simulink model "GPS1_Kvaser_R2018a_v3_0719"  (R2018a)
settings: Solver=FixedStepAuto  StartTime=0.0  StopTime=inf  FixedStep=0.02  RelTol=1e-3
undefined symbols (not defined in the file): canChannel
libraries: dspinverses x11, canmsglib x6, canlib x4
(part 2 of 2)

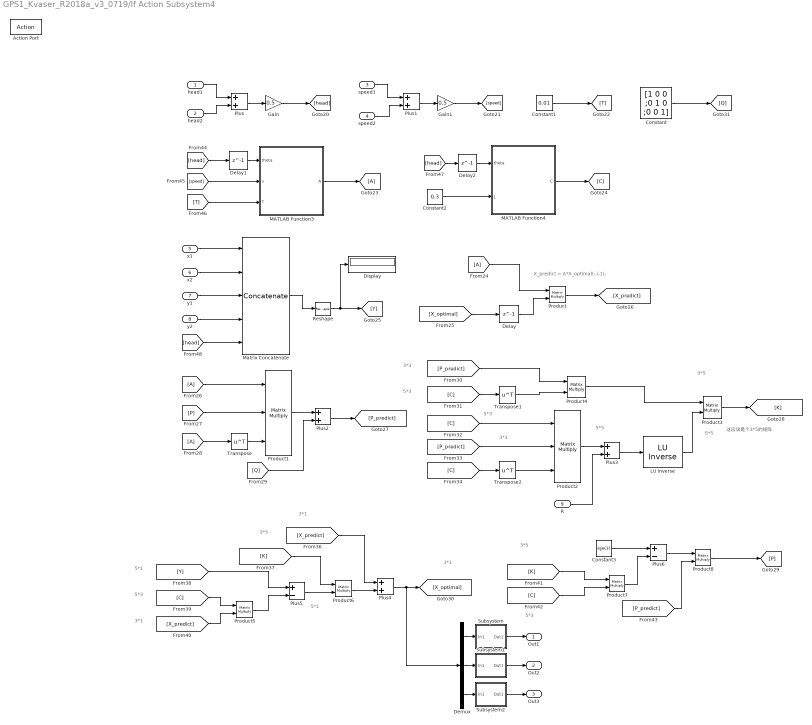
== system GPS1_Kvaser_R2018a_v3_0719/If Action Subsystem4 ==
  note: 5*3
  note: 这应该是个3*5的矩阵
  note: X_predict = A*X_optimal(:,i-1);
  note: 3*1
  note: 5*1
  note: 3*1
  note: 3*5
  note: 5*1
  note: 3*1
  note: 3*5
  note: 5*3
  note: 5*3
  note: 3*3
  note: 5*3
  note: 3*3
  note: 5*5
  note: 5*5
  note: 3*5
  head1 : Inport
  head2 : Inport  Port=2
  speed1 : Inport  Port=3
  speed2 : Inport  Port=4
  x1 : Inport  Port=5
  x2 : Inport  Port=6
  y1 : Inport  Port=7
  y2 : Inport  Port=8
  R : Inport  Port=9
  Action Port : ActionPort
  " LU Inverse" : dspinverses/ LU Inverse
  Constant : Constant  Value=[1 0 0 ;0 1 0 ;0 0 1]
  Constant1 : Constant  Value=0.01
  Constant2 : Constant  Value=0.3
  Constant3 : Constant  Value=eye(3)
  Delay : Delay  DelayLength=1
  Delay1 : Delay  DelayLength=1
  Delay2 : Delay  DelayLength=1
  Demux : Demux  Outputs=3
  Display : Display
  Gain : Gain  Gain=0.5
  Gain1 : Gain  Gain=0.5
  MATLAB Function3 : MATLAB Function  TreatAsAtomicUnit=on
  MATLAB Function4 : MATLAB Function  TreatAsAtomicUnit=on
  Matrix Concatenate : Concatenate  NumInputs=5  Mode=Multidimensional array  ConcatenateDimension=2
  Plus{,1..4} (5 alike) : Sum
  Plus5 : Sum  Inputs=+-
  Plus6 : Sum  Inputs=+-
  Product{,3..8} (7 alike) : Product  Multiplication=Matrix(*)
  Product1 : Product  Inputs=3  Multiplication=Matrix(*)
  Product2 : Product  Inputs=3  Multiplication=Matrix(*)
  Reshape : Reshape  OutputDimensionality=Customize  OutputDimensions=[5,1]
  Subsystem : Subsystem
  Subsystem1 : Subsystem
  Subsystem2 : Subsystem
  Transpose : Math  Operator=transpose  SaturateOnIntegerOverflow=on
  Transpose1 : Math  Operator=transpose  SaturateOnIntegerOverflow=on
  Transpose2 : Math  Operator=transpose  SaturateOnIntegerOverflow=on
  Out1 : Outport
  Out2 : Outport  Port=2
  Out3 : Outport  Port=3
  wires:
  x2/1 -> Matrix Concatenate/2
  y2/1 -> Matrix Concatenate/4
  head1/1 -> Plus/1
  Subsystem2/1(Out1) -> Out3/1
  speed2/1 -> Plus1/2
  x1/1 -> Matrix Concatenate/1
  speed1/1 -> Plus1/1
  head2/1 -> Plus/2
  Demux/1 -> Subsystem/1(In1)
  Demux/3 -> Subsystem2/1(In1)
  [T] -> MATLAB Function3/3(T)
  Product7/1 -> Plus6/2
  Plus/1 -> Gain/1
  [C] -> Product2/1
  [speed] -> MATLAB Function3/2(v)
  Transpose2/1 -> Product2/3
  Reshape/1 -> [Y], Display/1
  Matrix Concatenate/1 -> Reshape/1
  [X_predict] -> Product5/2
  [head] -> Delay2/1
  Transpose/1 -> Product1/3
  Plus1/1 -> Gain1/1
  [P_predict] -> Product4/1
  Gain/1 -> [head]
  Transpose1/1 -> Product4/2
  Constant1/1 -> [T]
  Constant3/1 -> Plus6/1
  " LU Inverse"/1 -> Product3/2
  Product1/1 -> Plus2/1
  [Y] -> Plus5/1
  [A] -> Product/1
  Demux/2 -> Subsystem1/1(In1)
  [K] -> Product7/1
  [A] -> Product1/1
  [Q] -> Plus2/2
  Product2/1 -> Plus3/1
  [head] -> Delay1/1
  [P_predict] -> Product8/2
  [P] -> Product1/2
  [X_predict] -> Plus4/1
  Plus3/1 -> " LU Inverse"/1
  [K] -> Product6/1
  Product3/1 -> [K]
  Plus2/1 -> [P_predict]
  [C] -> Product5/1
  R/1 -> Plus3/2
  Product6/1 -> Plus4/2
  [C] -> Transpose1/1
  [X_optimal] -> Delay/1
  Subsystem1/1(Out1) -> Out2/1
  MATLAB Function4/1(C) -> [C]
  Product5/1 -> Plus5/2
  Product/1 -> [X_predict]
  Product4/1 -> Product3/1
  Plus4/1 -> Demux/1, [X_optimal]
  Constant/1 -> [Q]
  [A] -> Transpose/1
  MATLAB Function3/1(A) -> [A]
  Constant2/1 -> MATLAB Function4/2(L)
  Delay/1 -> Product/2
  Product8/1 -> [P]
  Subsystem/1(Out1) -> Out1/1
  [C] -> Product7/2
  Plus6/1 -> Product8/1
  Plus5/1 -> Product6/2
  y1/1 -> Matrix Concatenate/3
  Gain1/1 -> [speed]
  [head] -> Matrix Concatenate/5
  [C] -> Transpose2/1
  [P_predict] -> Product2/2
  Delay1/1 -> MATLAB Function3/1(theta)
  Delay2/1 -> MATLAB Function4/1(theta)

== system GPS1_Kvaser_R2018a_v3_0719/If Action Subsystem5 ==
  In1 : Inport
  In2 : Inport  Port=2
  In3 : Inport  Port=3
  Action Port : ActionPort
  Out1 : Outport
  Out2 : Outport  Port=2
  Out3 : Outport  Port=3
  wires:
  In1/1 -> Out1/1
  In2/1 -> Out2/1
  In3/1 -> Out3/1

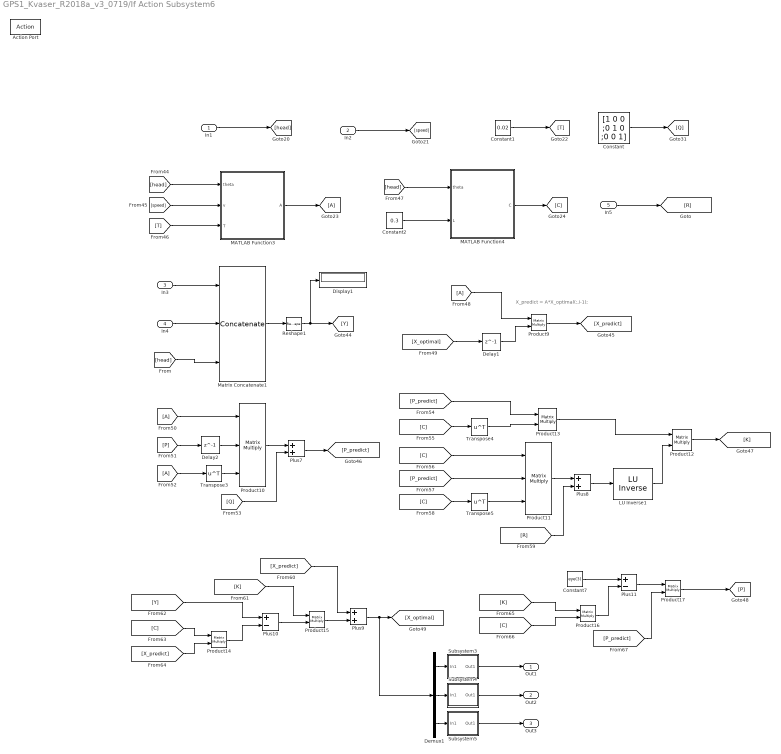
== system GPS1_Kvaser_R2018a_v3_0719/If Action Subsystem6 ==
  note: X_predict = A*X_optimal(:,i-1);
  In1 : Inport
  In2 : Inport  Port=2
  In3 : Inport  Port=3
  In4 : Inport  Port=4
  In5 : Inport  Port=5
  Action Port : ActionPort
  " LU Inverse1" : dspinverses/ LU Inverse
  Constant : Constant  Value=[1 0 0 ;0 1 0 ;0 0 1]
  Constant1 : Constant  Value=0.02
  Constant2 : Constant  Value=0.3
  Constant7 : Constant  Value=eye(3)
  Delay1 : Delay  DelayLength=1
  Delay2 : Delay  DelayLength=1
  Demux1 : Demux  Outputs=3
  Display1 : Display
  MATLAB Function3 : MATLAB Function  TreatAsAtomicUnit=on
  MATLAB Function4 : MATLAB Function  TreatAsAtomicUnit=on
  Matrix Concatenate1 : Concatenate  NumInputs=3  Mode=Multidimensional array  ConcatenateDimension=2
  Plus10 : Sum  Inputs=+-
  Plus11 : Sum  Inputs=+-
  Plus7 : Sum
  Plus8 : Sum
  Plus9 : Sum
  Product10 : Product  Inputs=3  Multiplication=Matrix(*)
  Product11 : Product  Inputs=3  Multiplication=Matrix(*)
  Product{9,12..17} (7 alike) : Product  Multiplication=Matrix(*)
  Reshape1 : Reshape  OutputDimensionality=Customize  OutputDimensions=[3,1]
  Subsystem3 : Subsystem
  Subsystem4 : Subsystem
  Subsystem5 : Subsystem
  Transpose3 : Math  Operator=transpose  SaturateOnIntegerOverflow=on
  Transpose4 : Math  Operator=transpose  SaturateOnIntegerOverflow=on
  Transpose5 : Math  Operator=transpose  SaturateOnIntegerOverflow=on
  Out1 : Outport
  Out2 : Outport  Port=2
  Out3 : Outport  Port=3
  wires:
  [head] -> MATLAB Function4/1(theta)
  Constant1/1 -> [T]
  [speed] -> MATLAB Function3/2(v)
  Subsystem5/1(Out1) -> Out3/1
  [head] -> MATLAB Function3/1(theta)
  Subsystem4/1(Out1) -> Out2/1
  [head] -> Matrix Concatenate1/3
  MATLAB Function3/1(A) -> [A]
  Subsystem3/1(Out1) -> Out1/1
  In4/1 -> Matrix Concatenate1/2
  Product9/1 -> [X_predict]
  [P_predict] -> Product11/2
  [K] -> Product15/1
  Product15/1 -> Plus9/2
  [X_optimal] -> Delay1/1
  [C] -> Product16/2
  Product13/1 -> Product12/1
  Demux1/3 -> Subsystem5/1(In1)
  [C] -> Transpose4/1
  Product12/1 -> [K]
  Transpose3/1 -> Product10/3
  [C] -> Transpose5/1
  [Y] -> Plus10/1
  Product17/1 -> [P]
  Matrix Concatenate1/1 -> Reshape1/1
  [A] -> Transpose3/1
  Transpose4/1 -> Product13/2
  In1/1 -> [head]
  Plus7/1 -> [P_predict]
  [A] -> Product9/1
  In5/1 -> [R]
  [C] -> Product11/1
  Constant2/1 -> MATLAB Function4/2(L)
  MATLAB Function4/1(C) -> [C]
  " LU Inverse1"/1 -> Product12/2
  Transpose5/1 -> Product11/3
  [X_predict] -> Product14/2
  Delay1/1 -> Product9/2
  Plus8/1 -> " LU Inverse1"/1
  [A] -> Product10/1
  Plus10/1 -> Product15/2
  Product11/1 -> Plus8/1
  [K] -> Product16/1
  [R] -> Plus8/2
  [P_predict] -> Product17/2
  [Q] -> Plus7/2
  [P_predict] -> Product13/1
  [C] -> Product14/1
  In2/1 -> [speed]
  Demux1/1 -> Subsystem3/1(In1)
  Reshape1/1 -> [Y], Display1/1
  [X_predict] -> Plus9/1
  Plus9/1 -> Demux1/1, [X_optimal]
  In3/1 -> Matrix Concatenate1/1
  Product14/1 -> Plus10/2
  Constant7/1 -> Plus11/1
  [T] -> MATLAB Function3/3(T)
  Product16/1 -> Plus11/2
  Plus11/1 -> Product17/1
  [P] -> Delay2/1
  Demux1/2 -> Subsystem4/1(In1)
  Constant/1 -> [Q]
  Product10/1 -> Plus7/1
  Delay2/1 -> Product10/2

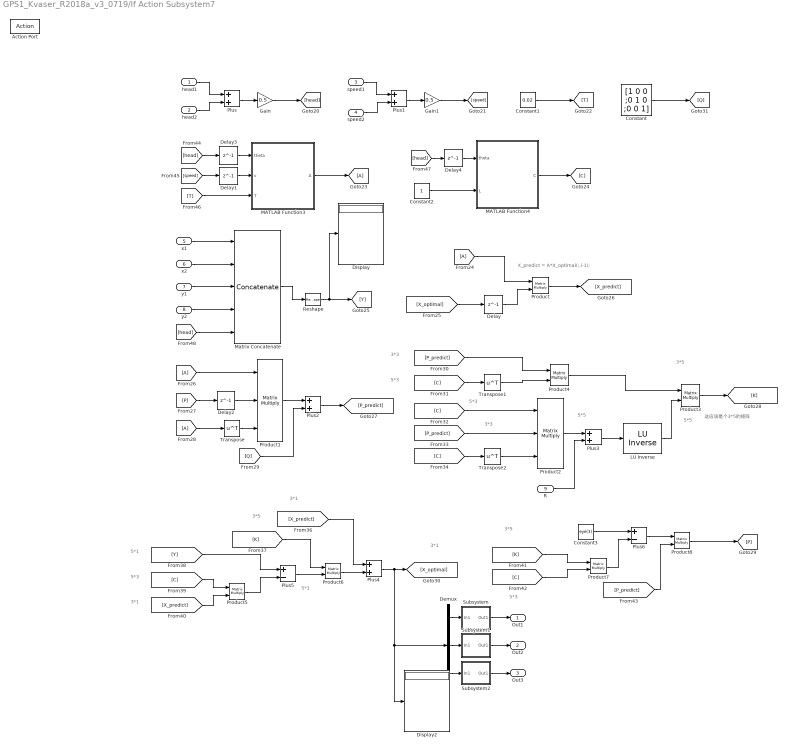
== system GPS1_Kvaser_R2018a_v3_0719/If Action Subsystem7 ==
  note: 5*3
  note: 这应该是个3*5的矩阵
  note: X_predict = A*X_optimal(:,i-1);
  note: 3*1
  note: 5*1
  note: 3*1
  note: 3*5
  note: 5*1
  note: 3*1
  note: 3*5
  note: 5*3
  note: 5*3
  note: 3*3
  note: 5*3
  note: 3*3
  note: 5*5
  note: 5*5
  note: 3*5
  head1 : Inport
  head2 : Inport  Port=2
  speed1 : Inport  Port=3
  speed2 : Inport  Port=4
  x1 : Inport  Port=5
  x2 : Inport  Port=6
  y1 : Inport  Port=7
  y2 : Inport  Port=8
  R : Inport  Port=9
  Action Port : ActionPort
  " LU Inverse" : dspinverses/ LU Inverse
  Constant : Constant  Value=[1 0 0 ;0 1 0 ;0 0 1]
  Constant1 : Constant  Value=0.02
  Constant2 : Constant
  Constant3 : Constant  Value=eye(3)
  Delay{,1..4} (5 alike) : Delay  DelayLength=1
  Demux : Demux  Outputs=3
  Display : Display
  Display2 : Display
  Gain : Gain  Gain=0.5
  Gain1 : Gain  Gain=0.5
  MATLAB Function3 : MATLAB Function  TreatAsAtomicUnit=on
  MATLAB Function4 : MATLAB Function  TreatAsAtomicUnit=on
  Matrix Concatenate : Concatenate  NumInputs=5  Mode=Multidimensional array  ConcatenateDimension=2
  Plus{,1..4} (5 alike) : Sum
  Plus5 : Sum  Inputs=+-
  Plus6 : Sum  Inputs=+-
  Product{,3..8} (7 alike) : Product  Multiplication=Matrix(*)
  Product1 : Product  Inputs=3  Multiplication=Matrix(*)
  Product2 : Product  Inputs=3  Multiplication=Matrix(*)
  Reshape : Reshape  OutputDimensionality=Customize  OutputDimensions=[5,1]
  Subsystem : Subsystem
  Subsystem1 : Subsystem
  Subsystem2 : Subsystem
  Transpose : Math  Operator=transpose  SaturateOnIntegerOverflow=on
  Transpose1 : Math  Operator=transpose  SaturateOnIntegerOverflow=on
  Transpose2 : Math  Operator=transpose  SaturateOnIntegerOverflow=on
  Out1 : Outport
  Out2 : Outport  Port=2
  Out3 : Outport  Port=3
  wires:
  x2/1 -> Matrix Concatenate/2
  y2/1 -> Matrix Concatenate/4
  head1/1 -> Plus/1
  Subsystem2/1(Out1) -> Out3/1
  speed2/1 -> Plus1/2
  x1/1 -> Matrix Concatenate/1
  speed1/1 -> Plus1/1
  head2/1 -> Plus/2
  Demux/1 -> Subsystem/1(In1)
  Demux/3 -> Subsystem2/1(In1)
  [T] -> MATLAB Function3/3(T)
  Product7/1 -> Plus6/2
  Plus/1 -> Gain/1
  [C] -> Product2/1
  [speed] -> Delay1/1
  Transpose2/1 -> Product2/3
  Reshape/1 -> [Y], Display/1
  Matrix Concatenate/1 -> Reshape/1
  [X_predict] -> Product5/2
  Transpose/1 -> Product1/3
  Plus1/1 -> Gain1/1
  [P_predict] -> Product4/1
  Gain/1 -> [head]
  Transpose1/1 -> Product4/2
  Constant1/1 -> [T]
  Constant3/1 -> Plus6/1
  " LU Inverse"/1 -> Product3/2
  Product1/1 -> Plus2/1
  [Y] -> Plus5/1
  [A] -> Product/1
  Demux/2 -> Subsystem1/1(In1)
  [K] -> Product7/1
  [A] -> Product1/1
  [Q] -> Plus2/2
  Product2/1 -> Plus3/1
  [P_predict] -> Product8/2
  [X_predict] -> Plus4/1
  Plus3/1 -> " LU Inverse"/1
  [K] -> Product6/1
  Product3/1 -> [K]
  Plus2/1 -> [P_predict]
  [C] -> Product5/1
  R/1 -> Plus3/2
  Product6/1 -> Plus4/2
  [C] -> Transpose1/1
  [X_optimal] -> Delay/1
  Subsystem1/1(Out1) -> Out2/1
  MATLAB Function4/1(C) -> [C]
  Product5/1 -> Plus5/2
  Product/1 -> [X_predict]
  Product4/1 -> Product3/1
  Plus4/1 -> Display2/1, Demux/1, [X_optimal]
  Constant/1 -> [Q]
  [A] -> Transpose/1
  MATLAB Function3/1(A) -> [A]
  Constant2/1 -> MATLAB Function4/2(L)
  Delay/1 -> Product/2
  Product8/1 -> [P]
  Subsystem/1(Out1) -> Out1/1
  [C] -> Product7/2
  Plus6/1 -> Product8/1
  Plus5/1 -> Product6/2
  y1/1 -> Matrix Concatenate/3
  Gain1/1 -> [speed]
  [head] -> Matrix Concatenate/5
  [C] -> Transpose2/1
  [P_predict] -> Product2/2
  [head] -> Delay3/1
  [head] -> Delay4/1
  [P] -> Delay2/1
  Delay1/1 -> MATLAB Function3/2(v)
  Delay3/1 -> MATLAB Function3/1(theta)
  Delay4/1 -> MATLAB Function4/1(theta)
  Delay2/1 -> Product1/2

== system GPS1_Kvaser_R2018a_v3_0719/If Action Subsystem8 ==
  In1 : Inport
  In2 : Inport  Port=2
  In3 : Inport  Port=3
  Action Port : ActionPort
  Out1 : Outport
  Out2 : Outport  Port=2
  Out3 : Outport  Port=3
  wires:
  In1/1 -> Out1/1
  In2/1 -> Out2/1
  In3/1 -> Out3/1

== system GPS1_Kvaser_R2018a_v3_0719/Subsystem ==
  In1 : Inport
  Delay : Delay  DelayLength=1
  Gain : Gain  Gain=0.1
  Gain1 : Gain  Gain=0.9
  Plus : Sum
  Out1 : Outport
  wires:
  In1/1 -> Gain/1
  Gain/1 -> Plus/1
  Plus/1 -> Delay/1, Out1/1
  Delay/1 -> Gain1/1
  Gain1/1 -> Plus/2

== system GPS1_Kvaser_R2018a_v3_0719/Subsystem1 ==
  In1 : Inport
  Delay : Delay  DelayLength=1
  Gain : Gain  Gain=0.1
  Gain1 : Gain  Gain=0.9
  Plus : Sum
  Out1 : Outport
  wires:
  Gain1/1 -> Plus/2
  Delay/1 -> Gain1/1
  Plus/1 -> Out1/1, Delay/1
  Gain/1 -> Plus/1
  In1/1 -> Gain/1

== system GPS1_Kvaser_R2018a_v3_0719/Subsystem2 ==
  In1 : Inport
  Delay : Delay  DelayLength=1
  Gain : Gain  Gain=0.1
  Gain1 : Gain  Gain=0.9
  Plus : Sum
  Out1 : Outport
  wires:
  In1/1 -> Gain/1
  Gain/1 -> Plus/1
  Plus/1 -> Delay/1, Out1/1
  Delay/1 -> Gain1/1
  Gain1/1 -> Plus/2

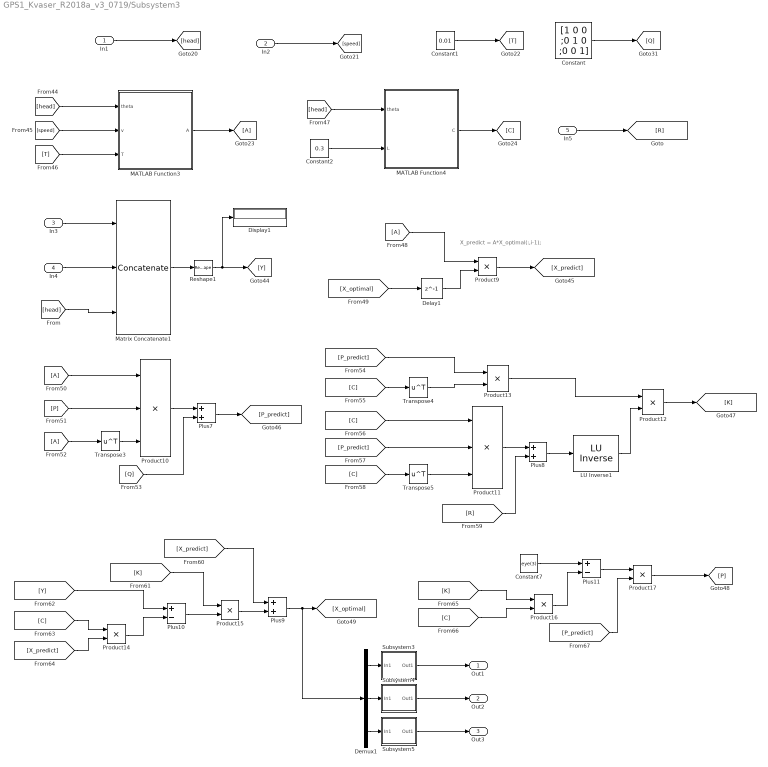
== system GPS1_Kvaser_R2018a_v3_0719/Subsystem3 ==
  note: X_predict = A*X_optimal(:,i-1);
  In1 : Inport
  In2 : Inport  Port=2
  In3 : Inport  Port=3
  In4 : Inport  Port=4
  In5 : Inport  Port=5
  " LU Inverse1" : dspinverses/ LU Inverse
  Constant : Constant  Value=[1 0 0 ;0 1 0 ;0 0 1]
  Constant1 : Constant  Value=0.01
  Constant2 : Constant  Value=0.3
  Constant7 : Constant  Value=eye(3)
  Delay1 : Delay  DelayLength=1
  Demux1 : Demux  Outputs=3
  Display1 : Display
  MATLAB Function3 : MATLAB Function  TreatAsAtomicUnit=on
  MATLAB Function4 : MATLAB Function  TreatAsAtomicUnit=on
  Matrix Concatenate1 : Concatenate  NumInputs=3  Mode=Multidimensional array  ConcatenateDimension=2
  Plus10 : Sum  Inputs=+-
  Plus11 : Sum  Inputs=+-
  Plus7 : Sum
  Plus8 : Sum
  Plus9 : Sum
  Product10 : Product  Inputs=3
  Product11 : Product  Inputs=3
  Product{9,12..17} (7 alike) : Product
  Reshape1 : Reshape  OutputDimensionality=Customize  OutputDimensions=[3,1]
  Subsystem3 : Subsystem
  Subsystem4 : Subsystem
  Subsystem5 : Subsystem
  Transpose3 : Math  Operator=transpose  SaturateOnIntegerOverflow=on
  Transpose4 : Math  Operator=transpose  SaturateOnIntegerOverflow=on
  Transpose5 : Math  Operator=transpose  SaturateOnIntegerOverflow=on
  Out1 : Outport
  Out2 : Outport  Port=2
  Out3 : Outport  Port=3
  wires:
  Product12/1 -> [K]
  [Y] -> Plus10/1
  Product17/1 -> [P]
  Transpose3/1 -> Product10/3
  [C] -> Transpose5/1
  Demux1/3 -> Subsystem5/1(In1)
  Product13/1 -> Product12/1
  Demux1/2 -> Subsystem4/1(In1)
  [C] -> Transpose4/1
  Plus10/1 -> Product15/2
  [C] -> Product16/2
  [X_optimal] -> Delay1/1
  [R] -> Plus8/2
  [P_predict] -> Product11/2
  Product9/1 -> [X_predict]
  [K] -> Product15/1
  Product15/1 -> Plus9/2
  Product10/1 -> Plus7/1
  Plus11/1 -> Product17/1
  [P] -> Product10/2
  Product16/1 -> Plus11/2
  Product14/1 -> Plus10/2
  Plus9/1 -> Demux1/1, [X_optimal]
  [X_predict] -> Plus9/1
  [C] -> Product14/1
  Demux1/1 -> Subsystem3/1(In1)
  Subsystem3/1(Out1) -> Out1/1
  Reshape1/1 -> [Y], Display1/1
  Subsystem5/1(Out1) -> Out3/1
  [P_predict] -> Product13/1
  [Q] -> Plus7/2
  Subsystem4/1(Out1) -> Out2/1
  [P_predict] -> Product17/2
  Product11/1 -> Plus8/1
  [K] -> Product16/1
  [A] -> Product10/1
  Constant7/1 -> Plus11/1
  Plus8/1 -> " LU Inverse1"/1
  Delay1/1 -> Product9/2
  [X_predict] -> Product14/2
  " LU Inverse1"/1 -> Product12/2
  Transpose5/1 -> Product11/3
  Transpose4/1 -> Product13/2
  Plus7/1 -> [P_predict]
  Matrix Concatenate1/1 -> Reshape1/1
  [C] -> Product11/1
  [A] -> Transpose3/1
  [A] -> Product9/1
  [T] -> MATLAB Function3/3(T)
  MATLAB Function3/1(A) -> [A]
  Constant/1 -> [Q]
  Constant2/1 -> MATLAB Function4/2(L)
  [head] -> MATLAB Function3/1(theta)
  [speed] -> MATLAB Function3/2(v)
  Constant1/1 -> [T]
  MATLAB Function4/1(C) -> [C]
  [head] -> MATLAB Function4/1(theta)
  In2/1 -> [speed]
  In1/1 -> [head]
  In4/1 -> Matrix Concatenate1/2
  In3/1 -> Matrix Concatenate1/1
  [head] -> Matrix Concatenate1/3
  In5/1 -> [R]

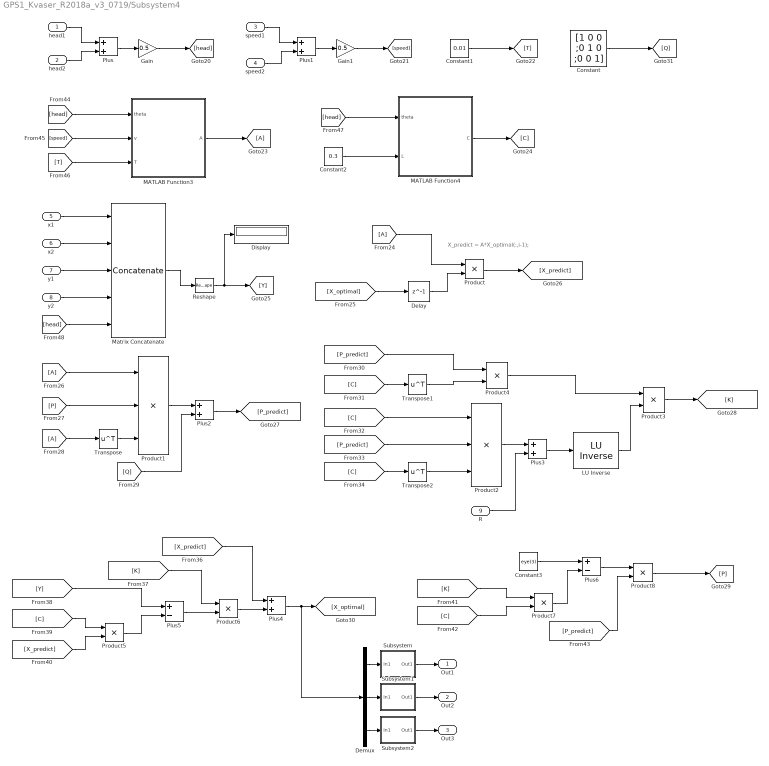
== system GPS1_Kvaser_R2018a_v3_0719/Subsystem4 ==
  note: X_predict = A*X_optimal(:,i-1);
  head1 : Inport
  head2 : Inport  Port=2
  speed1 : Inport  Port=3
  speed2 : Inport  Port=4
  x1 : Inport  Port=5
  x2 : Inport  Port=6
  y1 : Inport  Port=7
  y2 : Inport  Port=8
  R : Inport  Port=9
  " LU Inverse" : dspinverses/ LU Inverse
  Constant : Constant  Value=[1 0 0 ;0 1 0 ;0 0 1]
  Constant1 : Constant  Value=0.01
  Constant2 : Constant  Value=0.3
  Constant3 : Constant  Value=eye(3)
  Delay : Delay  DelayLength=1
  Demux : Demux  Outputs=3
  Display : Display
  Gain : Gain  Gain=0.5
  Gain1 : Gain  Gain=0.5
  MATLAB Function3 : MATLAB Function  TreatAsAtomicUnit=on
  MATLAB Function4 : MATLAB Function  TreatAsAtomicUnit=on
  Matrix Concatenate : Concatenate  NumInputs=5  Mode=Multidimensional array  ConcatenateDimension=2
  Plus{,1..4} (5 alike) : Sum
  Plus5 : Sum  Inputs=+-
  Plus6 : Sum  Inputs=+-
  Product{,3..8} (7 alike) : Product
  Product1 : Product  Inputs=3
  Product2 : Product  Inputs=3
  Reshape : Reshape  OutputDimensionality=Customize  OutputDimensions=[4,1]
  Subsystem : Subsystem
  Subsystem1 : Subsystem
  Subsystem2 : Subsystem
  Transpose : Math  Operator=transpose  SaturateOnIntegerOverflow=on
  Transpose1 : Math  Operator=transpose  SaturateOnIntegerOverflow=on
  Transpose2 : Math  Operator=transpose  SaturateOnIntegerOverflow=on
  Out1 : Outport
  Out2 : Outport  Port=2
  Out3 : Outport  Port=3
  wires:
  Subsystem1/1(Out1) -> Out2/1
  Subsystem/1(Out1) -> Out1/1
  [head] -> Matrix Concatenate/5
  Demux/1 -> Subsystem/1(In1)
  Demux/3 -> Subsystem2/1(In1)
  Demux/2 -> Subsystem1/1(In1)
  [T] -> MATLAB Function3/3(T)
  MATLAB Function4/1(C) -> [C]
  MATLAB Function3/1(A) -> [A]
  Constant/1 -> [Q]
  Constant2/1 -> MATLAB Function4/2(L)
  Product8/1 -> [P]
  [C] -> Transpose2/1
  Plus6/1 -> Product8/1
  [C] -> Product7/2
  Product4/1 -> Product3/1
  Product3/1 -> [K]
  Plus4/1 -> Demux/1, [X_optimal]
  [C] -> Product5/1
  [K] -> Product6/1
  [X_predict] -> Plus4/1
  [X_optimal] -> Delay/1
  Product6/1 -> Plus4/2
  head1/1 -> Plus/1
  [Y] -> Plus5/1
  Product1/1 -> Plus2/1
  [P_predict] -> Product8/2
  [P] -> Product1/2
  [Q] -> Plus2/2
  Product2/1 -> Plus3/1
  [K] -> Product7/1
  speed1/1 -> Plus1/1
  [P_predict] -> Product2/2
  speed2/1 -> Plus1/2
  y2/1 -> Matrix Concatenate/4
  R/1 -> Plus3/2
  Plus3/1 -> " LU Inverse"/1
  " LU Inverse"/1 -> Product3/2
  Constant3/1 -> Plus6/1
  x2/1 -> Matrix Concatenate/2
  [A] -> Product1/1
  Subsystem2/1(Out1) -> Out3/1
  Transpose/1 -> Product1/3
  [P_predict] -> Product4/1
  Transpose1/1 -> Product4/2
  Delay/1 -> Product/2
  Constant1/1 -> [T]
  y1/1 -> Matrix Concatenate/3
  [C] -> Transpose1/1
  Plus2/1 -> [P_predict]
  head2/1 -> Plus/2
  [C] -> Product2/1
  Transpose2/1 -> Product2/3
  [speed] -> MATLAB Function3/2(v)
  Gain1/1 -> [speed]
  Plus1/1 -> Gain1/1
  [X_predict] -> Product5/2
  Matrix Concatenate/1 -> Reshape/1
  Product5/1 -> Plus5/2
  Product7/1 -> Plus6/2
  Product/1 -> [X_predict]
  [A] -> Product/1
  Gain/1 -> [head]
  x1/1 -> Matrix Concatenate/1
  [A] -> Transpose/1
  [head] -> MATLAB Function3/1(theta)
  [head] -> MATLAB Function4/1(theta)
  Plus/1 -> Gain/1
  Reshape/1 -> [Y], Display/1
  Plus5/1 -> Product6/2

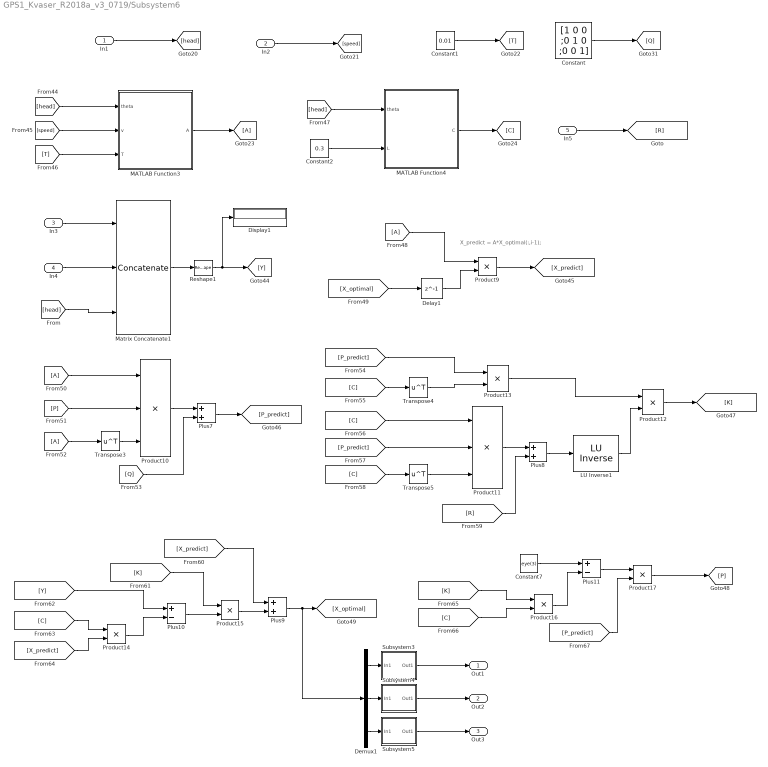
== system GPS1_Kvaser_R2018a_v3_0719/Subsystem6 ==
  note: X_predict = A*X_optimal(:,i-1);
  In1 : Inport
  In2 : Inport  Port=2
  In3 : Inport  Port=3
  In4 : Inport  Port=4
  In5 : Inport  Port=5
  " LU Inverse1" : dspinverses/ LU Inverse
  Constant : Constant  Value=[1 0 0 ;0 1 0 ;0 0 1]
  Constant1 : Constant  Value=0.01
  Constant2 : Constant  Value=0.3
  Constant7 : Constant  Value=eye(3)
  Delay1 : Delay  DelayLength=1
  Demux1 : Demux  Outputs=3
  Display1 : Display
  MATLAB Function3 : MATLAB Function  TreatAsAtomicUnit=on
  MATLAB Function4 : MATLAB Function  TreatAsAtomicUnit=on
  Matrix Concatenate1 : Concatenate  NumInputs=3  Mode=Multidimensional array  ConcatenateDimension=2
  Plus10 : Sum  Inputs=+-
  Plus11 : Sum  Inputs=+-
  Plus7 : Sum
  Plus8 : Sum
  Plus9 : Sum
  Product10 : Product  Inputs=3
  Product11 : Product  Inputs=3
  Product{9,12..17} (7 alike) : Product
  Reshape1 : Reshape  OutputDimensionality=Customize  OutputDimensions=[3,1]
  Subsystem3 : Subsystem
  Subsystem4 : Subsystem
  Subsystem5 : Subsystem
  Transpose3 : Math  Operator=transpose  SaturateOnIntegerOverflow=on
  Transpose4 : Math  Operator=transpose  SaturateOnIntegerOverflow=on
  Transpose5 : Math  Operator=transpose  SaturateOnIntegerOverflow=on
  Out1 : Outport
  Out2 : Outport  Port=2
  Out3 : Outport  Port=3
  wires:
  Product12/1 -> [K]
  [Y] -> Plus10/1
  Product17/1 -> [P]
  Transpose3/1 -> Product10/3
  [C] -> Transpose5/1
  Demux1/3 -> Subsystem5/1(In1)
  Product13/1 -> Product12/1
  Demux1/2 -> Subsystem4/1(In1)
  [C] -> Transpose4/1
  Plus10/1 -> Product15/2
  [C] -> Product16/2
  [X_optimal] -> Delay1/1
  [R] -> Plus8/2
  [P_predict] -> Product11/2
  Product9/1 -> [X_predict]
  [K] -> Product15/1
  Product15/1 -> Plus9/2
  Product10/1 -> Plus7/1
  Plus11/1 -> Product17/1
  [P] -> Product10/2
  Product16/1 -> Plus11/2
  Product14/1 -> Plus10/2
  Plus9/1 -> Demux1/1, [X_optimal]
  [X_predict] -> Plus9/1
  [C] -> Product14/1
  Demux1/1 -> Subsystem3/1(In1)
  Subsystem3/1(Out1) -> Out1/1
  Reshape1/1 -> [Y], Display1/1
  Subsystem5/1(Out1) -> Out3/1
  [P_predict] -> Product13/1
  [Q] -> Plus7/2
  Subsystem4/1(Out1) -> Out2/1
  [P_predict] -> Product17/2
  Product11/1 -> Plus8/1
  [K] -> Product16/1
  [A] -> Product10/1
  Constant7/1 -> Plus11/1
  Plus8/1 -> " LU Inverse1"/1
  Delay1/1 -> Product9/2
  [X_predict] -> Product14/2
  " LU Inverse1"/1 -> Product12/2
  Transpose5/1 -> Product11/3
  Transpose4/1 -> Product13/2
  Plus7/1 -> [P_predict]
  Matrix Concatenate1/1 -> Reshape1/1
  [C] -> Product11/1
  [A] -> Transpose3/1
  [A] -> Product9/1
  [T] -> MATLAB Function3/3(T)
  MATLAB Function3/1(A) -> [A]
  Constant/1 -> [Q]
  Constant2/1 -> MATLAB Function4/2(L)
  [head] -> MATLAB Function3/1(theta)
  [speed] -> MATLAB Function3/2(v)
  Constant1/1 -> [T]
  MATLAB Function4/1(C) -> [C]
  [head] -> MATLAB Function4/1(theta)
  In2/1 -> [speed]
  In1/1 -> [head]
  In4/1 -> Matrix Concatenate1/2
  In3/1 -> Matrix Concatenate1/1
  [head] -> Matrix Concatenate1/3
  In5/1 -> [R]

== system GPS1_Kvaser_R2018a_v3_0719/If Action Subsystem1/Subsystem3 ==
  In1 : Inport
  Delay : Delay  DelayLength=1
  Gain : Gain  Gain=0.1
  Gain1 : Gain  Gain=0.9
  Plus : Sum
  Out1 : Outport
  wires:
  In1/1 -> Gain/1
  Gain/1 -> Plus/1
  Plus/1 -> Delay/1, Out1/1
  Delay/1 -> Gain1/1
  Gain1/1 -> Plus/2

== system GPS1_Kvaser_R2018a_v3_0719/If Action Subsystem1/Subsystem4 ==
  In1 : Inport
  Delay : Delay  DelayLength=1
  Gain : Gain  Gain=0.1
  Gain1 : Gain  Gain=0.9
  Plus : Sum
  Out1 : Outport
  wires:
  Gain1/1 -> Plus/2
  Delay/1 -> Gain1/1
  Plus/1 -> Out1/1, Delay/1
  Gain/1 -> Plus/1
  In1/1 -> Gain/1

== system GPS1_Kvaser_R2018a_v3_0719/If Action Subsystem1/Subsystem5 ==
  In1 : Inport
  Delay : Delay  DelayLength=1
  Gain : Gain  Gain=0.1
  Gain1 : Gain  Gain=0.9
  Plus : Sum
  Out1 : Outport
  wires:
  In1/1 -> Gain/1
  Gain/1 -> Plus/1
  Plus/1 -> Delay/1, Out1/1
  Delay/1 -> Gain1/1
  Gain1/1 -> Plus/2

== system GPS1_Kvaser_R2018a_v3_0719/If Action Subsystem2/Subsystem3 ==
  In1 : Inport
  Delay : Delay  DelayLength=1
  Gain : Gain  Gain=0.1
  Gain1 : Gain  Gain=0.9
  Plus : Sum
  Out1 : Outport
  wires:
  In1/1 -> Gain/1
  Gain/1 -> Plus/1
  Plus/1 -> Delay/1, Out1/1
  Delay/1 -> Gain1/1
  Gain1/1 -> Plus/2

== system GPS1_Kvaser_R2018a_v3_0719/If Action Subsystem2/Subsystem4 ==
  In1 : Inport
  Delay : Delay  DelayLength=1
  Gain : Gain  Gain=0.1
  Gain1 : Gain  Gain=0.9
  Plus : Sum
  Out1 : Outport
  wires:
  Gain1/1 -> Plus/2
  Delay/1 -> Gain1/1
  Plus/1 -> Out1/1, Delay/1
  Gain/1 -> Plus/1
  In1/1 -> Gain/1

== system GPS1_Kvaser_R2018a_v3_0719/If Action Subsystem2/Subsystem5 ==
  In1 : Inport
  Delay : Delay  DelayLength=1
  Gain : Gain  Gain=0.1
  Gain1 : Gain  Gain=0.9
  Plus : Sum
  Out1 : Outport
  wires:
  In1/1 -> Gain/1
  Gain/1 -> Plus/1
  Plus/1 -> Delay/1, Out1/1
  Delay/1 -> Gain1/1
  Gain1/1 -> Plus/2

== system GPS1_Kvaser_R2018a_v3_0719/If Action Subsystem3/Subsystem3 ==
  In1 : Inport
  Delay : Delay  DelayLength=1
  Gain : Gain  Gain=0.1
  Gain1 : Gain  Gain=0.9
  Plus : Sum
  Out1 : Outport
  wires:
  In1/1 -> Gain/1
  Gain/1 -> Plus/1
  Plus/1 -> Delay/1, Out1/1
  Delay/1 -> Gain1/1
  Gain1/1 -> Plus/2

== system GPS1_Kvaser_R2018a_v3_0719/If Action Subsystem3/Subsystem4 ==
  In1 : Inport
  Delay : Delay  DelayLength=1
  Gain : Gain  Gain=0.1
  Gain1 : Gain  Gain=0.9
  Plus : Sum
  Out1 : Outport
  wires:
  Gain1/1 -> Plus/2
  Delay/1 -> Gain1/1
  Plus/1 -> Out1/1, Delay/1
  Gain/1 -> Plus/1
  In1/1 -> Gain/1

== system GPS1_Kvaser_R2018a_v3_0719/If Action Subsystem3/Subsystem5 ==
  In1 : Inport
  Delay : Delay  DelayLength=1
  Gain : Gain  Gain=0.1
  Gain1 : Gain  Gain=0.9
  Plus : Sum
  Out1 : Outport
  wires:
  In1/1 -> Gain/1
  Gain/1 -> Plus/1
  Plus/1 -> Delay/1, Out1/1
  Delay/1 -> Gain1/1
  Gain1/1 -> Plus/2

== system GPS1_Kvaser_R2018a_v3_0719/If Action Subsystem4/Subsystem ==
  In1 : Inport
  Delay : Delay  DelayLength=1
  Gain : Gain  Gain=0.1
  Gain1 : Gain  Gain=0.9
  Plus : Sum
  Out1 : Outport
  wires:
  In1/1 -> Gain/1
  Gain/1 -> Plus/1
  Plus/1 -> Delay/1, Out1/1
  Delay/1 -> Gain1/1
  Gain1/1 -> Plus/2

== system GPS1_Kvaser_R2018a_v3_0719/If Action Subsystem4/Subsystem1 ==
  In1 : Inport
  Delay : Delay  DelayLength=1
  Gain : Gain  Gain=0.1
  Gain1 : Gain  Gain=0.9
  Plus : Sum
  Out1 : Outport
  wires:
  Gain1/1 -> Plus/2
  Delay/1 -> Gain1/1
  Plus/1 -> Out1/1, Delay/1
  Gain/1 -> Plus/1
  In1/1 -> Gain/1

== system GPS1_Kvaser_R2018a_v3_0719/If Action Subsystem4/Subsystem2 ==
  In1 : Inport
  Delay : Delay  DelayLength=1
  Gain : Gain  Gain=0.1
  Gain1 : Gain  Gain=0.9
  Plus : Sum
  Out1 : Outport
  wires:
  In1/1 -> Gain/1
  Gain/1 -> Plus/1
  Plus/1 -> Delay/1, Out1/1
  Delay/1 -> Gain1/1
  Gain1/1 -> Plus/2

== system GPS1_Kvaser_R2018a_v3_0719/If Action Subsystem6/Subsystem3 ==
  In1 : Inport
  Delay : Delay  DelayLength=1
  Gain : Gain  Gain=0.1
  Gain1 : Gain  Gain=0.9
  Plus : Sum
  Out1 : Outport
  wires:
  In1/1 -> Gain/1
  Gain/1 -> Plus/1
  Plus/1 -> Delay/1, Out1/1
  Delay/1 -> Gain1/1
  Gain1/1 -> Plus/2

== system GPS1_Kvaser_R2018a_v3_0719/If Action Subsystem6/Subsystem4 ==
  In1 : Inport
  Delay : Delay  DelayLength=1
  Gain : Gain  Gain=0.1
  Gain1 : Gain  Gain=0.9
  Plus : Sum
  Out1 : Outport
  wires:
  Gain1/1 -> Plus/2
  Delay/1 -> Gain1/1
  Plus/1 -> Out1/1, Delay/1
  Gain/1 -> Plus/1
  In1/1 -> Gain/1

== system GPS1_Kvaser_R2018a_v3_0719/If Action Subsystem6/Subsystem5 ==
  In1 : Inport
  Delay : Delay  DelayLength=1
  Gain : Gain  Gain=0.1
  Gain1 : Gain  Gain=0.9
  Plus : Sum
  Out1 : Outport
  wires:
  In1/1 -> Gain/1
  Gain/1 -> Plus/1
  Plus/1 -> Delay/1, Out1/1
  Delay/1 -> Gain1/1
  Gain1/1 -> Plus/2

== system GPS1_Kvaser_R2018a_v3_0719/If Action Subsystem7/Subsystem ==
  In1 : Inport
  Delay : Delay  DelayLength=1
  Gain : Gain  Gain=0.1
  Gain1 : Gain  Gain=0.9
  Plus : Sum
  Out1 : Outport
  wires:
  In1/1 -> Gain/1
  Gain/1 -> Plus/1
  Plus/1 -> Delay/1, Out1/1
  Delay/1 -> Gain1/1
  Gain1/1 -> Plus/2

== system GPS1_Kvaser_R2018a_v3_0719/If Action Subsystem7/Subsystem1 ==
  In1 : Inport
  Delay : Delay  DelayLength=1
  Gain : Gain  Gain=0.1
  Gain1 : Gain  Gain=0.9
  Plus : Sum
  Out1 : Outport
  wires:
  Gain1/1 -> Plus/2
  Delay/1 -> Gain1/1
  Plus/1 -> Out1/1, Delay/1
  Gain/1 -> Plus/1
  In1/1 -> Gain/1

== system GPS1_Kvaser_R2018a_v3_0719/If Action Subsystem7/Subsystem2 ==
  In1 : Inport
  Delay : Delay  DelayLength=1
  Gain : Gain  Gain=0.1
  Gain1 : Gain  Gain=0.9
  Plus : Sum
  Out1 : Outport
  wires:
  In1/1 -> Gain/1
  Gain/1 -> Plus/1
  Plus/1 -> Delay/1, Out1/1
  Delay/1 -> Gain1/1
  Gain1/1 -> Plus/2

== system GPS1_Kvaser_R2018a_v3_0719/Subsystem3/Subsystem3 ==
  In1 : Inport
  Delay : Delay  DelayLength=1
  Gain : Gain  Gain=0.1
  Gain1 : Gain  Gain=0.9
  Plus : Sum
  Out1 : Outport
  wires:
  In1/1 -> Gain/1
  Gain/1 -> Plus/1
  Plus/1 -> Delay/1, Out1/1
  Delay/1 -> Gain1/1
  Gain1/1 -> Plus/2

== system GPS1_Kvaser_R2018a_v3_0719/Subsystem3/Subsystem4 ==
  In1 : Inport
  Delay : Delay  DelayLength=1
  Gain : Gain  Gain=0.1
  Gain1 : Gain  Gain=0.9
  Plus : Sum
  Out1 : Outport
  wires:
  Gain1/1 -> Plus/2
  Delay/1 -> Gain1/1
  Plus/1 -> Out1/1, Delay/1
  Gain/1 -> Plus/1
  In1/1 -> Gain/1

== system GPS1_Kvaser_R2018a_v3_0719/Subsystem3/Subsystem5 ==
  In1 : Inport
  Delay : Delay  DelayLength=1
  Gain : Gain  Gain=0.1
  Gain1 : Gain  Gain=0.9
  Plus : Sum
  Out1 : Outport
  wires:
  In1/1 -> Gain/1
  Gain/1 -> Plus/1
  Plus/1 -> Delay/1, Out1/1
  Delay/1 -> Gain1/1
  Gain1/1 -> Plus/2

== system GPS1_Kvaser_R2018a_v3_0719/Subsystem4/Subsystem ==
  In1 : Inport
  Delay : Delay  DelayLength=1
  Gain : Gain  Gain=0.1
  Gain1 : Gain  Gain=0.9
  Plus : Sum
  Out1 : Outport
  wires:
  In1/1 -> Gain/1
  Gain/1 -> Plus/1
  Plus/1 -> Delay/1, Out1/1
  Delay/1 -> Gain1/1
  Gain1/1 -> Plus/2

== system GPS1_Kvaser_R2018a_v3_0719/Subsystem4/Subsystem1 ==
  In1 : Inport
  Delay : Delay  DelayLength=1
  Gain : Gain  Gain=0.1
  Gain1 : Gain  Gain=0.9
  Plus : Sum
  Out1 : Outport
  wires:
  Gain1/1 -> Plus/2
  Delay/1 -> Gain1/1
  Plus/1 -> Out1/1, Delay/1
  Gain/1 -> Plus/1
  In1/1 -> Gain/1

== system GPS1_Kvaser_R2018a_v3_0719/Subsystem4/Subsystem2 ==
  In1 : Inport
  Delay : Delay  DelayLength=1
  Gain : Gain  Gain=0.1
  Gain1 : Gain  Gain=0.9
  Plus : Sum
  Out1 : Outport
  wires:
  In1/1 -> Gain/1
  Gain/1 -> Plus/1
  Plus/1 -> Delay/1, Out1/1
  Delay/1 -> Gain1/1
  Gain1/1 -> Plus/2

== system GPS1_Kvaser_R2018a_v3_0719/Subsystem6/Subsystem3 ==
  In1 : Inport
  Delay : Delay  DelayLength=1
  Gain : Gain  Gain=0.1
  Gain1 : Gain  Gain=0.9
  Plus : Sum
  Out1 : Outport
  wires:
  In1/1 -> Gain/1
  Gain/1 -> Plus/1
  Plus/1 -> Delay/1, Out1/1
  Delay/1 -> Gain1/1
  Gain1/1 -> Plus/2

== system GPS1_Kvaser_R2018a_v3_0719/Subsystem6/Subsystem4 ==
  In1 : Inport
  Delay : Delay  DelayLength=1
  Gain : Gain  Gain=0.1
  Gain1 : Gain  Gain=0.9
  Plus : Sum
  Out1 : Outport
  wires:
  Gain1/1 -> Plus/2
  Delay/1 -> Gain1/1
  Plus/1 -> Out1/1, Delay/1
  Gain/1 -> Plus/1
  In1/1 -> Gain/1

== system GPS1_Kvaser_R2018a_v3_0719/Subsystem6/Subsystem5 ==
  In1 : Inport
  Delay : Delay  DelayLength=1
  Gain : Gain  Gain=0.1
  Gain1 : Gain  Gain=0.9
  Plus : Sum
  Out1 : Outport
  wires:
  In1/1 -> Gain/1
  Gain/1 -> Plus/1
  Plus/1 -> Delay/1, Out1/1
  Delay/1 -> Gain1/1
  Gain1/1 -> Plus/2

== matlab function GPS1_Kvaser_R2018a_v3_0719/MATLAB Function1 ==
  data: EKF_mode output; sate1 input; sate2 input
function EKF_mode = fcn(sate1,sate2)
if sate1 < 4 && sate2 >= 4
%     R  = [1 0 0 ;
%         0 1 0 ;
%         0 0 1 ;];
    EKF_mode = 3;
elseif sate1 >= 4 && sate2 < 4
%     R  = [1 0 0 ;
%         0 1 0 ;
%         0 0 1 ;];
    EKF_mode = 2;
elseif sate1 >= 4 && sate2 >= 4
%     R = [13-sate1 0 0 0 0 ;
%         0 13-sate1 0 0 0 ;
%         0 0 13-sate2 0 0 ;
%         0 0 0 13-sate2 0 ;
%         0 0 0 0 13-max(sate1,sate2);];
    EKF_mode = 1;
else
%     R = zeros(5,5);
    EKF_mode = 0;
end

== matlab function GPS1_Kvaser_R2018a_v3_0719/MATLAB Function ==
  data: dikaerY1 output; dikaerY2 output; lat1 input; dikaerX1 output; lat2 input; long1 input; long2 input; dikaerX2 output
function [dikaerY1,dikaerY2,dikaerX1,dikaerX2] = long_lat(lat1,lat2,long1,long2)
M_PI=3.14159265358979323846;
L = 6381372 * M_PI * 2;
W = L;
H = L / 2;
mill = 2.3;
n = length(long1);
% x1 = long1 * M_PI / 180;
% y1 = lat1 * M_PI / 180;
% y1 = 1.25 * log(tan(0.25 * M_PI + 0.4 * y1));
% dikaerX1 = (W / 2) + (W / (2 * M_PI)) * x1 ;
% dikaerY1 = (H / 2) - (H / (2 * mill)) * y1 ;
% x2 = long2 * M_PI / 180;
% y2 = lat2 * M_PI / 180;
% y2 = 1.25 * log(tan(0.25 * M_PI + 0.4 * y2));
% dikaerX2 = (W / 2) + (W / (2 * M_PI)) * x2 ;
% dikaerY2 = (H / 2) - (H / (2 * mill)) * y2 ;

x1 = long1 * M_PI / 180;
y1 = lat1 * M_PI / 180;
y1 = 1.25 * log(tan(0.25 * M_PI + 0.4 * y1));
dikaerX1 = (W / 2) + (W / (2 * M_PI)) * x1  - 3.33571*10^7;
dikaerY1 = (H / 2) - (H / (2 * mill)) * y1 -6.81892*10^6;
x2 = long2 * M_PI / 180;
y2 = lat2 * M_PI / 180;
y2 = 1.25 * log(tan(0.25 * M_PI + 0.4 * y2));
dikaerX2 = (W / 2) + (W / (2 * M_PI)) * x2 - 3.33571*10^7;
dikaerY2 = (H / 2) - (H / (2 * mill)) * y2 - 6.81892*10^6;

== matlab function GPS1_Kvaser_R2018a_v3_0719/Subsystem6/MATLAB Function3 ==
  data: theta input; A output; v input; T input
function A = fcn(theta,v,T)
A = [1 0 -T*v*sin(theta);0 1 T*v*cos(theta);0 0 1]
end

== matlab function GPS1_Kvaser_R2018a_v3_0719/MATLAB Function3 ==
  data: theta input; A output; v input; T input
function A = fcn(theta,v,T)
A = [1 0 -T*v*sin(theta);0 1 T*v*cos(theta);0 0 1]
end

== matlab function GPS1_Kvaser_R2018a_v3_0719/MATLAB Function4 ==
  data: theta input; C output; L input
function C = fcn(theta,L)
C = [1 0 L/2*sin(theta);1 0 -L/2*sin(theta);0 1 -L/2*cos(theta);0 1 -L/2*cos(theta);0 0 1];
end

== matlab function GPS1_Kvaser_R2018a_v3_0719/Subsystem6/MATLAB Function4 ==
  data: theta input; C output; L input
function C = fcn(theta,L)
C = [1 0 L/2*sin(theta);1 0 -L/2*sin(theta);0 1 -L/2*cos(theta);0 1 -L/2*cos(theta);0 0 1];
end

== matlab function GPS1_Kvaser_R2018a_v3_0719/Subsystem3/MATLAB Function3 ==
  data: theta input; A output; v input; T input
function A = fcn(theta,v,T)
A = [1 0 -T*v*sin(theta);0 1 T*v*cos(theta);0 0 1]
end

== matlab function GPS1_Kvaser_R2018a_v3_0719/Subsystem3/MATLAB Function4 ==
  data: theta input; C output; L input
function C = fcn(theta,L)
C = [1 0 L/2*sin(theta);1 0 -L/2*sin(theta);0 1 -L/2*cos(theta);0 1 -L/2*cos(theta);0 0 1];
end

== matlab function GPS1_Kvaser_R2018a_v3_0719/Subsystem4/MATLAB Function3 ==
  data: theta input; A output; v input; T input
function A = fcn(theta,v,T)
A = [1 0 -T*v*sin(theta);0 1 T*v*cos(theta);0 0 1]
end

== matlab function GPS1_Kvaser_R2018a_v3_0719/Subsystem4/MATLAB Function4 ==
  data: theta input; C output; L input
function C = fcn(theta,L)
C = [1 0 L/2*sin(theta);1 0 -L/2*sin(theta);0 1 -L/2*cos(theta);0 1 -L/2*cos(theta);0 0 1];
end

== matlab function GPS1_Kvaser_R2018a_v3_0719/If Action Subsystem1/MATLAB Function3 ==
  data: theta input; A output; v input; T input
function A = fcn(theta,v,T)
A = [1 0 -T*v*sin(theta);0 1 T*v*cos(theta);0 0 1]
end

== matlab function GPS1_Kvaser_R2018a_v3_0719/If Action Subsystem1/MATLAB Function4 ==
  data: theta input; C output; L input
function C = fcn(theta,L)
C = [
    1 0 -L/2*sin(theta);
    
    0 1 -L/2*cos(theta);
    0 0 1];
end

== matlab function GPS1_Kvaser_R2018a_v3_0719/If Action Subsystem4/MATLAB Function3 ==
  data: theta input; A output; v input; T input
function A = fcn(theta,v,T)
A = [1 0 -T*v*sin(theta);
    0 1 T*v*cos(theta);
    0 0 1]
end

== matlab function GPS1_Kvaser_R2018a_v3_0719/If Action Subsystem4/MATLAB Function4 ==
  data: theta input; C output; L input
function C = fcn(theta,L)
C=zeros(5,3);
C = [1 0 L/2*sin(theta);
    1 0 -L/2*sin(theta);
    0 1 -L/2*cos(theta);
    0 1 -L/2*cos(theta);
    0 0 1];

== matlab function GPS1_Kvaser_R2018a_v3_0719/If Action Subsystem3/MATLAB Function3 ==
  data: theta input; A output; v input; T input
function A = fcn(theta,v,T)
A = [1 0 -T*v*sin(theta);0 1 T*v*cos(theta);0 0 1]
end

== matlab function GPS1_Kvaser_R2018a_v3_0719/If Action Subsystem3/MATLAB Function4 ==
  data: theta input; C output; L input
function C = fcn(theta,L)
C = [1 0 L/2*sin(theta);
    %1 0 -L/2*sin(theta);
    0 1 -L/2*cos(theta);
    %0 1 -L/2*cos(theta);
    0 0 1];
end

== matlab function GPS1_Kvaser_R2018a_v3_0719/MATLAB Function2 ==
  data: sate1 input; R output; sate2 input
function R = fcn(sate1,sate2)
    R = [13-sate1 0 0 0 0 ;
        0 13-sate1 0 0 0 ;
        0 0 13-sate2 0 0 ;
        0 0 0 13-sate2 0 ;
        0 0 0 0 13-max(sate1,sate2);];

== matlab function GPS1_Kvaser_R2018a_v3_0719/If Action Subsystem2/MATLAB Function3 ==
  data: theta input; A output; v input; T input
function A = fcn(theta,v,T)
A = [1 0 -T*v*sin(theta);0 1 T*v*cos(theta);0 0 1]
end

== matlab function GPS1_Kvaser_R2018a_v3_0719/If Action Subsystem2/MATLAB Function4 ==
  data: theta input; C output; L input
function C = fcn(theta,L)
C = [
    1 0 -L/2*sin(theta);
    
    0 1 -L/2*cos(theta);
    0 0 1];
end

== matlab function GPS1_Kvaser_R2018a_v3_0719/If Action Subsystem6/MATLAB Function3 ==
  data: theta input; A output; v input; T input
function A = fcn(theta,v,T)
A = [1 0 -T*v*sin(theta);0 1 T*v*cos(theta);0 0 1]
end

== matlab function GPS1_Kvaser_R2018a_v3_0719/If Action Subsystem6/MATLAB Function4 ==
  data: theta input; C output; L input
function C = fcn(theta,L)
C = [1 0 L/2*sin(theta);
    %1 0 -L/2*sin(theta);
    0 1 -L/2*cos(theta);
    %0 1 -L/2*cos(theta);
    0 0 1];
end

== matlab function GPS1_Kvaser_R2018a_v3_0719/If Action Subsystem7/MATLAB Function3 ==
  data: theta input; A output; v input; T input
function A = fcn(theta,v,T)
% A = [1 0 -T*v*sin(theta);
%     0 1 T*v*cos(theta);
%     0 0 1];
A = [1 0 T*v*cos(theta);
    0 1 -T*v*sin(theta);
    0 0 1]
A = [1 0 0;
    0 1 -T*v*sin(theta);
    0 0 1]
end

== matlab function GPS1_Kvaser_R2018a_v3_0719/If Action Subsystem7/MATLAB Function4 ==
  data: theta input; C output; L input
function C = fcn(theta,L)
C=zeros(5,3);
C = [1 0 L/2*sin(theta);
    1 0 -L/2*sin(theta);
    0 1 -L/2*cos(theta);
    0 1 -L/2*cos(theta);
    0 0 1];
C = [1 0 -L/2*cos(theta);
    1 0 -L/2*cos(theta);
    0 1 L/2*sin(theta);
    0 1 -L/2*sin(theta);
    0 0 1];
C = [1 0 0;
    1 0 0;
    0 1 L/2*sin(theta);
    0 1 -L/2*sin(theta);
    0 0 1];

== matlab function GPS1_Kvaser_R2018a_v3_0719/MATLAB Function5 ==
  data: sate1 input; R output; sate2 input
function R = fcn(sate1,sate2)
    R = [13-sate1 0 0 0 0 ;
        0 13-sate1 0 0 0 ;
        0 0 13-sate2 0 0 ;
        0 0 0 13-sate2 0 ;
        0 0 0 0 13-max(sate1,sate2);];

== matlab function GPS1_Kvaser_R2018a_v3_0719/MATLAB Function6 ==
  data: kf_vehicle_speed input; speed_end output; speed1 input; speed2 input; sate1 input; sate2 input
function speed_end = fcn(kf_vehicle_speed,speed1,speed2,sate1,sate2)
sate1_rate = sate1/48;
sate2_rate = sate2/48;
speed_end = (sate1_rate*speed1+sate2_rate*speed2)+(1-sate1_rate-sate2_rate)*kf_vehicle_speed;
end

== matlab function GPS1_Kvaser_R2018a_v3_0719/MATLAB Function7 ==
  data: long1 input; lat1 input; A_x1 output; A_y1 output
function [A_x1,A_y1] = long_lat(long1,lat1)
M_PI=3.14159265358979323846;
L = 6381372 * M_PI * 2;
W = L;
H = L / 2;
mill = 2.3;
x1 = long1 * M_PI / 180;
y1 = lat1 * M_PI / 180;
y1_1 = 1.25 * log(tan(0.25 * M_PI + 0.4 * y1));
A_x1 = (W / 2) + (W / (2 * M_PI)) * x1 ;
A_y1 = (H / 2) - (H / (2 * mill)) * y1_1 ;
end
